simulink model "RajamaniController"  (R2018a)
settings: Solver=ode45  StartTime=0.0  StopTime=1  FixedStep=0.002  RelTol=1e-3  EnableMultiTasking=on
values from neighbouring files (symbols this model uses):
  A = [0 1 0 0; 0 A22 A23 A24; 0 0 0 1; 0 A42 A43 A44;]    [data.m]
  B1 = [0; B1_12; 0; B1_14]    [data.m]
  B2 = [0; B2_12; 0; B2_14]    [data.m]
  delta_ff = (L/R)+((Kv*ay)-(k3*e2_ss))    [data.m]
  K = place(A, B1, P)    [data.m]
  m = 1573    [data.m]
  PsiDot_des = Vx/R    (= 0.03)    [data.m]
undefined symbols (not defined in the file or in its folder): Bx_ash_f, Bx_ash_r, Bx_snow_f, Bx_snow_r, By_ash_f, By_ash_r, By_snow_f, By_snow_r, Cx_ash_f, Cx_ash_r, Cx_snow_f, Cx_snow_r, Cy_ash_f, Cy_ash_r, Cy_snow_f, Cy_snow_r, D_phi, D_theta, DELTA_OFFSET, delta_r, epsilon, Ex_ash_f, Ex_ash_r, Ex_snow_f, Ex_snow_r, Ey_ash_f, Ey_ash_r, Ey_snow_f, Ey_snow_r, g, h, Iw, Ixx, Iyy, Izz, K_phi, K_theta, l_f, l_r, mu_x_ash_f, mu_x_ash_r, mu_x_snow_f, mu_x_snow_r, mu_y_ash_f, mu_y_ash_r, mu_y_snow_f, mu_y_snow_r, omega0, road, Rw, Ts, Tsmall, Vx0, w
(part 2 of 2)

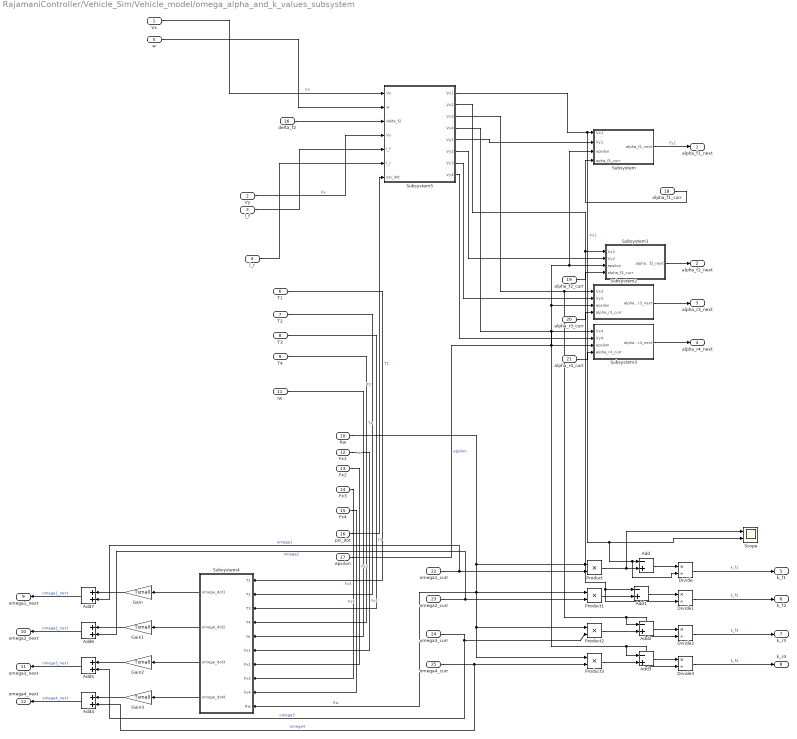
== system RajamaniController/Vehicle_Sim/Vehicle_model/omega_alpha_and_k_values_subsystem ==
  Vx : Inport  OutDataTypeStr=double  SampleTime=Ts
  Vy : Inport  Port=2  OutDataTypeStr=double  SampleTime=Ts
  l_f : Inport  Port=3  OutDataTypeStr=double  SampleTime=Ts
  l_r : Inport  Port=4  OutDataTypeStr=double  SampleTime=Ts
  w : Inport  Port=5  OutDataTypeStr=double  SampleTime=Ts
  T1 : Inport  Port=6  OutDataTypeStr=double  SampleTime=Ts
  T2 : Inport  Port=7  OutDataTypeStr=double  SampleTime=Ts
  T3 : Inport  Port=8  OutDataTypeStr=double  SampleTime=Ts
  T4 : Inport  Port=9  OutDataTypeStr=double  SampleTime=Ts
  Rw : Inport  Port=10  OutDataTypeStr=double  SampleTime=Ts
  Iw : Inport  Port=11  OutDataTypeStr=double  SampleTime=Ts
  Fx1 : Inport  Port=12  OutDataTypeStr=double  SampleTime=Ts
  Fx2 : Inport  Port=13  OutDataTypeStr=double  SampleTime=Ts
  Fx3 : Inport  Port=14  OutDataTypeStr=double  SampleTime=Ts
  Fx4 : Inport  Port=15  OutDataTypeStr=double  SampleTime=Ts
  psi_dot : Inport  Port=16  OutDataTypeStr=double  SampleTime=Ts
  epsilon : Inport  Port=17  OutDataTypeStr=double  SampleTime=Ts
  alpha_f1_curr : Inport  Port=18  OutDataTypeStr=double  SampleTime=Tsmall
  alpha_f2_curr : Inport  Port=19  OutDataTypeStr=double  SampleTime=Tsmall
  alpha_r3_curr : Inport  Port=20  OutDataTypeStr=double  SampleTime=Tsmall
  alpha_r4_curr : Inport  Port=21  OutDataTypeStr=double  SampleTime=Tsmall
  omega1_curr : Inport  Port=22  OutDataTypeStr=double  SampleTime=Ts
  omega2_curr : Inport  Port=23  OutDataTypeStr=double  SampleTime=Ts
  omega3_curr : Inport  Port=24  OutDataTypeStr=double  SampleTime=Ts
  omega4_curr : Inport  Port=25  OutDataTypeStr=double  SampleTime=Ts
  delta_f2 : Inport  Port=26  OutDataTypeStr=double  SampleTime=Ts
  Add{,1..3} (4 alike) : Sum  Inputs=-+
  Add{4..7} (4 alike) : Sum
  Divide{,1..3} (4 alike) : Product  Inputs=*/
  Gain{,1..3} (4 alike) : Gain  Gain=Tsmall
  Product{,1..3} (4 alike) : Product
  Scope : Scope  NumInputPorts=2
  Subsystem : Subsystem
  Subsystem1 : Subsystem
  Subsystem2 : Subsystem
  Subsystem3 : Subsystem
  Subsystem4 : Subsystem
  Subsystem5 : Subsystem
  alpha_f1_next : Outport  OutDataTypeStr=double  SampleTime=Ts
  alpha_f2_next : Outport  Port=2  OutDataTypeStr=double  SampleTime=Tsmall
  alpha_r3_next : Outport  Port=3  OutDataTypeStr=double  SampleTime=Tsmall
  alpha_r4_next : Outport  Port=4  OutDataTypeStr=double  SampleTime=Tsmall
  k_f1 : Outport  Port=5  OutDataTypeStr=double  SampleTime=Ts
  k_f2 : Outport  Port=6  OutDataTypeStr=double  SampleTime=Ts
  k_r3 : Outport  Port=7  OutDataTypeStr=double  SampleTime=Ts
  k_r4 : Outport  Port=8  OutDataTypeStr=double  SampleTime=Ts
  omega1_next : Outport  Port=9
  omega2_next : Outport  Port=10
  omega3_next : Outport  Port=11
  omega4_next : Outport  Port=12
  wires:
  Subsystem5/1(Vx1) -> Scope/2, Divide/2, Add/1, Subsystem/1(Vx1)  "Vx1"
  epsilon/1 -> Subsystem3/3(epsilon), Subsystem2/3(epsilon), Subsystem1/3(epsilon), Subsystem/3(epsilon)  "epsilon"
  Subsystem1/1(alpha_f2_next) -> alpha_f2_next/1
  Divide/1 -> k_f1/1  "k_f1"
  omega1_curr/1 -> Add7/2, Product/2  "omega1"
  omega2_curr/1 -> Add6/2, Product1/2  "omega2"
  omega3_curr/1 -> Add5/2, Product2/2  "omega3"
  omega4_curr/1 -> Add4/2, Product3/2  "omega4"
  Rw/1 -> Subsystem4/10(Rw), Product1/1, Product3/1, Product2/1, Product/1  "Rw"
  Product/1 -> Scope/1, Add/2
  Add/1 -> Divide/1
  Product1/1 -> Add1/2
  Add1/1 -> Divide1/1
  Product2/1 -> Add2/2
  Add2/1 -> Divide2/1
  Product3/1 -> Add3/2
  Add3/1 -> Divide3/1
  Divide1/1 -> k_f2/1  "k_f2"
  Divide2/1 -> k_r3/1  "k_f3"
  Divide3/1 -> k_r4/1  "k_f4"
  T1/1 -> Subsystem4/1(T1)  "T1"
  T2/1 -> Subsystem4/2(T2)  "T2"
  T3/1 -> Subsystem4/3(T3)  "T3"
  T4/1 -> Subsystem4/4(T4)  "T4"
  Iw/1 -> Subsystem4/5(Iw)  "Iw"
  Fx1/1 -> Subsystem4/6(Fx1)  "Fx1"
  Fx2/1 -> Subsystem4/7(Fx2)  "Fx2"
  Fx3/1 -> Subsystem4/8(Fx3)  "Fx3"
  Fx4/1 -> Subsystem4/9(Fx4)  "Fx4"
  Subsystem4/1(omega_dot1) -> Gain/1
  Subsystem4/2(omega_dot2) -> Gain1/1
  Subsystem4/3(omega_dot3) -> Gain2/1
  Subsystem4/4(omega_dot4) -> Gain3/1
  alpha_f1_curr/1 -> Subsystem/4(apha_f1_curr)
  alpha_f2_curr/1 -> Subsystem1/4(alpha_f2_curr)
  Subsystem2/1(alpha_r3_next) -> alpha_r3_next/1
  alpha_r3_curr/1 -> Subsystem2/4(alpha_r3_curr)
  Subsystem3/1(alpha_r4_next) -> alpha_r4_next/1
  alpha_r4_curr/1 -> Subsystem3/4(alpha_r4_curr)
  Gain1/1 -> Add6/1
  Gain/1 -> Add7/1
  Gain2/1 -> Add5/1
  Gain3/1 -> Add4/1
  Add7/1 -> omega1_next/1  "omega1_next"
  Add6/1 -> omega2_next/1  "omega2_next"
  Add5/1 -> omega3_next/1  "omega3_next"
  Add4/1 -> omega4_next/1  "omega4_next"
  Subsystem5/2(Vx2) -> Divide1/2, Add1/1, Subsystem1/1(Vx2)
  Subsystem5/4(Vx4) -> Subsystem3/1(Vx4), Add3/1, Divide3/2
  Subsystem5/3(Vx3) -> Subsystem2/1(Vx3), Add2/1, Divide2/2
  Vx/1 -> Subsystem5/1(Vx)  "Vx"
  w/1 -> Subsystem5/2(w)
  Vy/1 -> Subsystem5/4(Vy)  "Vy"
  l_f/1 -> Subsystem5/5(l_f)
  l_r/1 -> Subsystem5/6(l_r)
  psi_dot/1 -> Subsystem5/7(psi_dot)
  Subsystem5/5(Vy1) -> Subsystem/2(Vy1)
  Subsystem5/6(Vy2) -> Subsystem1/2(Vy2)
  Subsystem5/7(Vy3) -> Subsystem2/2(Vy3)
  Subsystem5/8(Vy4) -> Subsystem3/2(Vy4)
  delta_f2/1 -> Subsystem5/3(delta_f2)
  Subsystem/1(alpha_f1_next) -> alpha_f1_next/1  "Fy1"

== system RajamaniController/Vehicle_Sim/Vehicle_model/phi_subsystem ==
  FY : Inport  OutDataTypeStr=double  SampleTime=Ts
  psi_dot : Inport  Port=2  OutDataTypeStr=double  SampleTime=Tsmall
  phi_dot : Inport  Port=3  OutDataTypeStr=double  SampleTime=Tsmall
  phi : Inport  Port=4  OutDataTypeStr=double  SampleTime=Tsmall
  theta_dot : Inport  Port=5  OutDataTypeStr=double  SampleTime=Tsmall
  theta : Inport  Port=6  OutDataTypeStr=double  SampleTime=Tsmall
  Ixx : Inport  Port=7  OutDataTypeStr=double  SampleTime=Ts
  Iyy : Inport  Port=8  OutDataTypeStr=double  SampleTime=Ts
  Izz : Inport  Port=9  OutDataTypeStr=double  SampleTime=Ts
  K_phi : Inport  Port=10  OutDataTypeStr=double  SampleTime=Ts
  D_phi : Inport  Port=11  OutDataTypeStr=double  SampleTime=Ts
  h : Inport  Port=12  OutDataTypeStr=double  SampleTime=Ts
  Divide : Product  Inputs=*/
  phi_ddot_denominator_subsystem : Subsystem
  phi_ddot_numerator_subsystem : Subsystem
  phi_ddot : Outport  OutDataTypeStr=double  SampleTime=Tsmall
  wires:
  phi_ddot_numerator_subsystem/1(phi_ddot_numerator) -> Divide/1
  phi/1 -> phi_ddot_denominator_subsystem/1(phi), phi_ddot_numerator_subsystem/4(phi)
  FY/1 -> phi_ddot_numerator_subsystem/1(FY)
  theta_dot/1 -> phi_ddot_numerator_subsystem/5(theta_dot)
  phi_dot/1 -> phi_ddot_numerator_subsystem/3(phi_dot)
  theta/1 -> phi_ddot_numerator_subsystem/6(theta), phi_ddot_denominator_subsystem/2(theta)
  psi_dot/1 -> phi_ddot_numerator_subsystem/2(psi_dot)
  Divide/1 -> phi_ddot/1
  phi_ddot_denominator_subsystem/1(phi_ddot_denominator) -> Divide/2
  Ixx/1 -> phi_ddot_denominator_subsystem/3(Ixx)
  Iyy/1 -> phi_ddot_denominator_subsystem/4(Iyy), phi_ddot_numerator_subsystem/7(Iyy)
  Izz/1 -> phi_ddot_numerator_subsystem/8(Izz), phi_ddot_denominator_subsystem/5(Izz)
  K_phi/1 -> phi_ddot_numerator_subsystem/9(K_phi)
  D_phi/1 -> phi_ddot_numerator_subsystem/10(D_phi)
  h/1 -> phi_ddot_numerator_subsystem/11(h)

== system RajamaniController/Vehicle_Sim/Vehicle_model/psi_subsystem ==
  FX : Inport  OutDataTypeStr=double  SampleTime=Ts
  FY : Inport  Port=2  OutDataTypeStr=double  SampleTime=Ts
  MZ : Inport  Port=3  OutDataTypeStr=double  SampleTime=Ts
  phi : Inport  Port=4  OutDataTypeStr=double  SampleTime=Ts
  theta : Inport  Port=5  OutDataTypeStr=double  SampleTime=Ts
  Ixx : Inport  Port=6  OutDataTypeStr=double  SampleTime=Ts
  Iyy : Inport  Port=7  OutDataTypeStr=double  SampleTime=Ts
  Izz : Inport  Port=8  OutDataTypeStr=double  SampleTime=Ts
  h : Inport  Port=9  OutDataTypeStr=double  SampleTime=Ts
  Add : Sum
  Add1 : Sum  Inputs=+-
  Add2 : Sum
  Add3 : Sum
  Divide{,1..6,8} (8 alike) : Product  Inputs=**
  Divide7 : Product  Inputs=*/
  Square{,1..3} (4 alike) : Math  Operator=square  RndMeth=Zero  SaturateOnIntegerOverflow=on
  Trigonometric Function : Trigonometry
  Trigonometric Function1 : Trigonometry
  Trigonometric Function2 : Trigonometry  Operator=cos
  Trigonometric Function3 : Trigonometry  Operator=cos
  psi_ddot : Outport
  wires:
  Square/1 -> Divide3/1
  MZ/1 -> Add1/1
  Trigonometric Function2/1 -> Square2/1, Divide2/1
  Divide2/1 -> Add/2
  Ixx/1 -> Divide3/2
  Add2/1 -> Divide4/2
  Square2/1 -> Divide6/2
  Divide6/1 -> Add2/2
  Divide3/1 -> Add3/1
  Add3/1 -> Divide7/2
  FY/1 -> Divide1/1
  FX/1 -> Divide/1
  Trigonometric Function3/1 -> Square3/1
  Iyy/1 -> Divide5/1
  Divide1/1 -> Divide2/2
  Square3/1 -> Divide4/1
  Izz/1 -> Divide6/1
  Trigonometric Function/1 -> Square/1, Divide1/2
  Trigonometric Function1/1 -> Square1/1, Divide/2
  phi/1 -> Trigonometric Function1/1, Trigonometric Function2/1
  theta/1 -> Trigonometric Function3/1, Trigonometric Function/1
  Divide8/1 -> Add1/2
  Add/1 -> Divide8/1
  Divide5/1 -> Add2/1
  Add1/1 -> Divide7/1
  Divide/1 -> Add/1
  Divide7/1 -> psi_ddot/1  "psi_ddot"
  Divide4/1 -> Add3/2
  Square1/1 -> Divide5/2
  h/1 -> Divide8/2

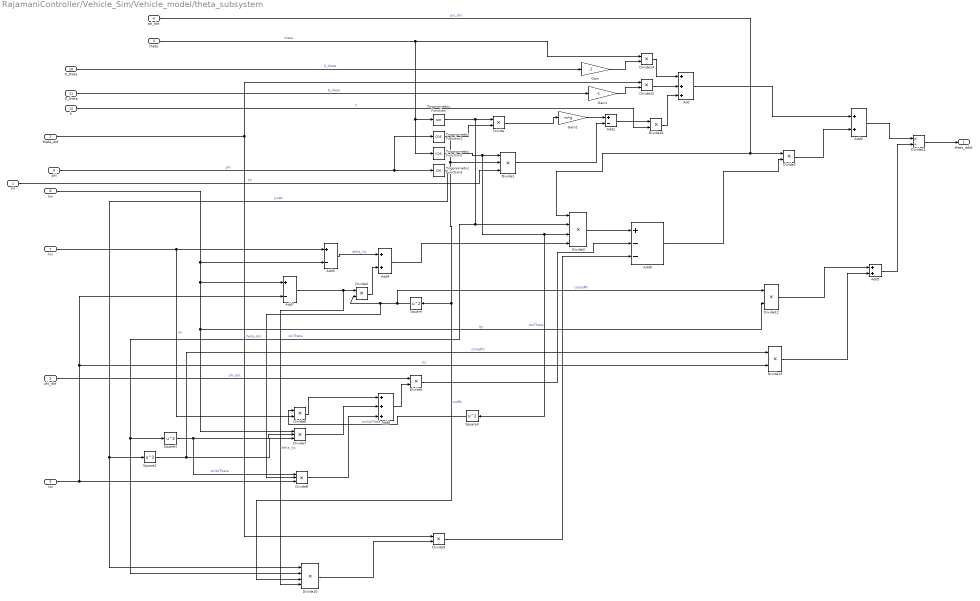
== system RajamaniController/Vehicle_Sim/Vehicle_model/theta_subsystem ==
  FX : Inport  OutDataTypeStr=double  SampleTime=Ts
  theta_dot : Inport  Port=2  OutDataTypeStr=double  SampleTime=Ts
  theta : Inport  Port=3  OutDataTypeStr=double  SampleTime=Ts
  psi_dot : Inport  Port=4  OutDataTypeStr=double  SampleTime=Ts
  phi_dot : Inport  Port=5  OutDataTypeStr=double  SampleTime=Ts
  phi : Inport  Port=6  OutDataTypeStr=double  SampleTime=Ts
  Ixx : Inport  Port=7  OutDataTypeStr=double  SampleTime=Ts
  Iyy : Inport  Port=8  OutDataTypeStr=double  SampleTime=Ts
  Izz : Inport  Port=9  OutDataTypeStr=double  SampleTime=Ts
  K_theta : Inport  Port=10  OutDataTypeStr=double  SampleTime=Ts
  D_theta : Inport  Port=11  OutDataTypeStr=double  SampleTime=Ts
  h : Inport  Port=12  OutDataTypeStr=double  SampleTime=Ts
  Add : Sum  Inputs=+++
  Add1 : Sum  Inputs=+-
  Add2 : Sum
  Add3 : Sum  Inputs=+-
  Add4 : Sum
  Add5 : Sum
  Add7 : Sum  Inputs=+-
  Add8 : Sum  Inputs=+++
  Add9 : Sum  Inputs=+--
  Divide{,2,4..6,9,12..16} (11 alike) : Product  Inputs=**
  Divide1 : Product  Inputs=***
  Divide10 : Product  Inputs=****
  Divide11 : Product  Inputs=*/
  Divide3 : Product  Inputs=****
  Divide7 : Product  Inputs=***
  Divide8 : Product  Inputs=***
  Gain : Gain  Gain=-1  OutDataTypeStr=double
  Gain1 : Gain  Gain=-1  OutDataTypeStr=double
  Gain2 : Gain  Gain=m*g  OutDataTypeStr=double
  Square{,1..3} (4 alike) : Math  Operator=square  RndMeth=Zero  SaturateOnIntegerOverflow=on
  Trigonometric Function : Trigonometry
  Trigonometric Function1 : Trigonometry  Operator=cos
  Trigonometric Function2 : Trigonometry  Operator=cos
  Trigonometric Function3 : Trigonometry
  theta_ddot : Outport  OutDataTypeStr=double  SampleTime=Tsmall
  wires:
  Add/1 -> Add2/1
  Divide8/1 -> Add8/3
  Add4/1 -> Divide3/4
  Divide1/1 -> Add1/2
  Add8/1 -> Divide5/2
  Add1/1 -> Divide16/1
  Square1/1 -> Divide8/1, Divide7/2  "sinSqTheta"
  Divide7/1 -> Add8/2
  Add9/1 -> Divide2/2
  Square/1 -> Divide12/1, Divide8/2, Divide4/2  "cosSqPhi"
  Trigonometric Function3/1 -> Divide10/1, Square2/1  "sinPhi"
  Gain2/1 -> Add1/1
  Square2/1 -> Divide13/1, Divide7/3  "sinSqPhi"
  Trigonometric Function2/1 -> Square3/1, Divide3/3, Divide1/1  "cosTheta"
  Divide/1 -> Gain2/1
  Divide10/1 -> Divide9/2
  Trigonometric Function/1 -> Divide10/2, Square1/1, Divide3/2, Divide/1  "sinTheta"
  Divide6/1 -> Add8/1
  Divide2/1 -> Add2/2
  Divide9/1 -> Add9/3
  Divide5/1 -> Add9/2
  Gain/1 -> Divide14/2
  Divide4/1 -> Add4/2
  Add3/1 -> Add4/1  "delta_Ixy"
  Divide3/1 -> Add9/1
  Trigonometric Function1/1 -> Divide10/3, Square/1, Divide1/2, Divide/2  "cosPhi"
  Add7/1 -> Divide10/4, Divide4/1  "delta_Iyz"
  Divide16/1 -> Add/3
  Gain1/1 -> Divide15/2
  theta/1 -> Divide14/1, Trigonometric Function/1, Trigonometric Function2/1  "theta"
  Iyy/1 -> Divide7/1, Divide12/2, Add7/1, Add3/2  "Iyy"
  phi_dot/1 -> Divide5/1  "phi_dot"
  Ixx/1 -> Add3/1, Divide6/2  "Ixx"
  FX/1 -> Divide1/3  "FX"
  theta_dot/1 -> Divide15/1, Divide9/1  "theta_dot"
  Izz/1 -> Divide13/2, Add7/2, Divide8/3  "Izz"
  phi/1 -> Trigonometric Function1/1, Trigonometric Function3/1  "phi"
  psi_dot/1 -> Divide3/1, Divide2/1  "psi_dot"
  Add2/1 -> Divide11/1
  Divide11/1 -> theta_ddot/1
  Add5/1 -> Divide11/2
  Divide12/1 -> Add5/1
  Divide13/1 -> Add5/2
  Divide15/1 -> Add/2
  Divide14/1 -> Add/1
  K_theta/1 -> Gain/1  "K_theta"
  D_theta/1 -> Gain1/1  "D_theta"
  h/1 -> Divide16/2  "h"
  Square3/1 -> Divide6/1  "cosSqTheta"

== system RajamaniController/Vehicle_Sim/Vehicle_model/Fz_Subsystem/tau_phi_subsystem ==
  K_phi : Inport
  D_phi : Inport  Port=2
  phi_dot : Inport  Port=3
  phi : Inport  Port=4
  Add : Sum
  Add1 : Sum
  Divide{,1..3} (4 alike) : Product  Inputs=**
  Gain : Gain  Gain=0.5
  Gain1 : Gain  Gain=0.5
  tau_phi_f : Outport
  tau_phi_r : Outport  Port=2
  wires:
  Divide2/1 -> Add1/1
  Divide/1 -> Add/1
  Add/1 -> tau_phi_f/1  "tau_phi_f"
  Divide1/1 -> Add/2
  Gain1/1 -> Divide3/1, Divide1/1  "D_phi_r"
  Gain/1 -> Divide2/1, Divide/1  "K_phi_r"
  D_phi/1 -> Gain1/1
  phi/1 -> Divide2/2, Divide/2  "phi"
  Divide3/1 -> Add1/2
  phi_dot/1 -> Divide3/2, Divide1/2  "phi_dot"
  K_phi/1 -> Gain/1
  Add1/1 -> tau_phi_r/1  "tau_phi_r"

== system RajamaniController/Vehicle_Sim/Vehicle_model/Fz_Subsystem/tau_theta_subsystem ==
  theta_dot : Inport  OutDataTypeStr=double  SampleTime=Ts  LockScale=on
  theta : Inport  Port=2  OutDataTypeStr=double  SampleTime=Ts
  K_theta : Inport  Port=3  OutDataTypeStr=double  SampleTime=Ts
  D_theta : Inport  Port=4  OutDataTypeStr=double  SampleTime=Ts
  Add : Sum
  Divide : Product  Inputs=**
  Divide1 : Product  Inputs=**
  tau_theta : Outport  OutDataTypeStr=double  SampleTime=Ts
  wires:
  Add/1 -> tau_theta/1
  Divide/1 -> Add/1
  Divide1/1 -> Add/2
  K_theta/1 -> Divide/1
  D_theta/1 -> Divide1/2
  theta_dot/1 -> Divide1/1
  theta/1 -> Divide/2

== system RajamaniController/Vehicle_Sim/Vehicle_model/Pacjeka_parameters_Subsystem/Ashphalt_condition_subsystem ==
  Action Port : ActionPort
  Bx_ash_f : Constant  Value=Bx_ash_f
  Bx_ash_r : Constant  Value=Bx_ash_r
  By_ash_f : Constant  Value=By_ash_f
  By_ash_r : Constant  Value=By_ash_r
  Cx_ash_f : Constant  Value=Cx_ash_f
  Cx_ash_r : Constant  Value=Cx_ash_r
  Cy_ash_f : Constant  Value=Cy_ash_f
  Cy_ash_r : Constant  Value=Cy_ash_r
  Ex_ash_f : Constant  Value=Ex_ash_f
  Ex_ash_r : Constant  Value=Ex_ash_r
  Ey_ash_f : Constant  Value=Ey_ash_f
  Ey_ash_r : Constant  Value=Ey_ash_r
  Mux : Mux  Inputs=16
      settings: DisplayOption=signals
  mu_x_ash_f : Constant  Value=mu_x_ash_f
  mu_x_ash_r : Constant  Value=mu_x_ash_r
  mu_y_ash_f : Constant  Value=mu_y_ash_f
  mu_y_ash_r : Constant  Value=mu_y_ash_r
  Out1 : Outport  OutDataTypeStr=double  SampleTime=Ts
  wires:
  mu_x_ash_f/1 -> Mux/1  "mu_x_ash_f"
  mu_y_ash_f/1 -> Mux/2  "mu_y_ash_f"
  Cx_ash_f/1 -> Mux/3  "Cx_ash_f"
  Cy_ash_f/1 -> Mux/4  "Cy_ash_f"
  Bx_ash_f/1 -> Mux/5  "Bx_ash_f"
  By_ash_f/1 -> Mux/6  "By_ash_f"
  Ex_ash_f/1 -> Mux/7  "Ex_ash_f"
  Ey_ash_f/1 -> Mux/8  "E_y_ash_f"
  Cy_ash_r/1 -> Mux/12  "Cy_ash_r"
  Cx_ash_r/1 -> Mux/11  "Cx_ash_r"
  By_ash_r/1 -> Mux/14  "By_ash_r"
  Bx_ash_r/1 -> Mux/13  "Bx_ash_r"
  mu_y_ash_r/1 -> Mux/10  "mu_y_ash_r"
  Ex_ash_r/1 -> Mux/15  "Ex_ash_r"
  mu_x_ash_r/1 -> Mux/9  "mu_x_ash_r"
  Ey_ash_r/1 -> Mux/16  "Ey_ash_r"
  Mux/1 -> Out1/1

== system RajamaniController/Vehicle_Sim/Vehicle_model/Pacjeka_parameters_Subsystem/Snow_condition_subsystem ==
  Action Port : ActionPort
  Bx_snow_f : Constant  Value=Bx_snow_f
  Bx_snow_r : Constant  Value=Bx_snow_r
  By_snow_f : Constant  Value=By_snow_f
  By_snow_r : Constant  Value=By_snow_r
  Cx_snow_f : Constant  Value=Cx_snow_f
  Cx_snow_r : Constant  Value=Cx_snow_r
  Cy_snow_f : Constant  Value=Cy_snow_f
  Cy_snow_r : Constant  Value=Cy_snow_r
  Ex_snow_f : Constant  Value=Ex_snow_f
  Ex_snow_r : Constant  Value=Ex_snow_r
  Ey_snow_f : Constant  Value=Ey_snow_f
  Ey_snow_r : Constant  Value=Ey_snow_r
  Mux : Mux  Inputs=16
  mu_x_snow_f : Constant  Value=mu_x_snow_f
  mu_x_snow_r : Constant  Value=mu_x_snow_r
  mu_y_snow_f : Constant  Value=mu_y_snow_f
  mu_y_snow_r : Constant  Value=mu_y_snow_r
  Out1 : Outport  OutDataTypeStr=double  SampleTime=Ts
  wires:
  Ex_snow_r/1 -> Mux/15
  Cy_snow_r/1 -> Mux/12
  By_snow_r/1 -> Mux/14
  Cx_snow_r/1 -> Mux/11
  mu_y_snow_r/1 -> Mux/10
  mu_x_snow_r/1 -> Mux/9
  Bx_snow_r/1 -> Mux/13
  Ey_snow_r/1 -> Mux/16
  mu_x_snow_f/1 -> Mux/1
  mu_y_snow_f/1 -> Mux/2
  Cx_snow_f/1 -> Mux/3
  Cy_snow_f/1 -> Mux/4
  Bx_snow_f/1 -> Mux/5
  By_snow_f/1 -> Mux/6
  Ex_snow_f/1 -> Mux/7
  Ey_snow_f/1 -> Mux/8
  Mux/1 -> Out1/1

== system RajamaniController/Vehicle_Sim/Vehicle_model/omega_alpha_and_k_values_subsystem/Subsystem ==
  Vx1 : Inport  OutDataTypeStr=double  SampleTime=Ts
  Vy1 : Inport  Port=2  OutDataTypeStr=double  SampleTime=Ts
  epsilon : Inport  Port=3  OutDataTypeStr=double  SampleTime=Ts
  apha_f1_curr : Inport  Port=4  OutDataTypeStr=double  SampleTime=Tsmall
  Add : Sum  Inputs=+-
  Add1 : Sum
  Divide : Product  Inputs=*/
  Divide1 : Product  Inputs=*/
  Gain : Gain  Gain=-1
  Gain1 : Gain  Gain=Tsmall
  Product : Product
  Product1 : Product
  Trigonometric Function : Trigonometry  Operator=atan
  alpha_f1_next : Outport  OutDataTypeStr=double  SampleTime=Tsmall
  wires:
  Gain1/1 -> Add1/1  "alpha_f1dot*Tsmall"
  Vx1/1 -> Divide1/2, Divide/1
  Product1/1 -> Add/2
  Divide1/1 -> Trigonometric Function/1
  Divide/1 -> Gain/1, Product1/1
  Product/1 -> Add/1
  epsilon/1 -> Divide/2
  Trigonometric Function/1 -> Product/2
  Vy1/1 -> Divide1/1
  Add/1 -> Gain1/1  "alpha_f1_dot"
  Gain/1 -> Product/1
  Add1/1 -> alpha_f1_next/1
  apha_f1_curr/1 -> Add1/2, Product1/2  "Fy1"

== system RajamaniController/Vehicle_Sim/Vehicle_model/omega_alpha_and_k_values_subsystem/Subsystem1 ==
  Vx2 : Inport  OutDataTypeStr=double  SampleTime=Ts
  Vy2 : Inport  Port=2  OutDataTypeStr=double  SampleTime=Ts
  epsilon : Inport  Port=3  OutDataTypeStr=double  SampleTime=Ts
  alpha_f2_curr : Inport  Port=4  OutDataTypeStr=double  SampleTime=Tsmall
  Add : Sum  Inputs=+-
  Add1 : Sum
  Divide : Product  Inputs=*/
  Divide1 : Product  Inputs=*/
  Gain : Gain  Gain=-1
  Gain1 : Gain  Gain=Tsmall
  Product : Product
  Product1 : Product
  Trigonometric Function : Trigonometry  Operator=atan
  alpha_f2_next : Outport  OutDataTypeStr=double  SampleTime=Tsmall
  wires:
  Gain1/1 -> Add1/1  "alpha_f2dot*Tsmall"
  Vx2/1 -> Divide1/2, Divide/1
  Product1/1 -> Add/2
  Divide1/1 -> Trigonometric Function/1
  Divide/1 -> Gain/1, Product1/1
  Product/1 -> Add/1
  epsilon/1 -> Divide/2
  Trigonometric Function/1 -> Product/2
  Vy2/1 -> Divide1/1
  Add/1 -> Gain1/1  "alpha_f2_dot"
  Gain/1 -> Product/1
  alpha_f2_curr/1 -> Add1/2, Product1/2
  Add1/1 -> alpha_f2_next/1

== system RajamaniController/Vehicle_Sim/Vehicle_model/omega_alpha_and_k_values_subsystem/Subsystem2 ==
  Vx3 : Inport  OutDataTypeStr=double  SampleTime=Ts
  Vy3 : Inport  Port=2  OutDataTypeStr=double  SampleTime=Ts
  epsilon : Inport  Port=3  OutDataTypeStr=double  SampleTime=Ts
  alpha_r3_curr : Inport  Port=4  OutDataTypeStr=double  SampleTime=Tsmall
  Add : Sum  Inputs=+-
  Add1 : Sum
  Divide : Product  Inputs=*/
  Divide1 : Product  Inputs=*/
  Gain : Gain  Gain=-1
  Gain1 : Gain  Gain=Tsmall
  Product : Product
  Product1 : Product
  Trigonometric Function : Trigonometry  Operator=atan
  alpha_r3_next : Outport  OutDataTypeStr=double  SampleTime=Tsmall
  wires:
  Gain1/1 -> Add1/1  "alpha_r3dot*Tsmall"
  Vx3/1 -> Divide1/2, Divide/1
  Product1/1 -> Add/2
  Divide1/1 -> Trigonometric Function/1
  Divide/1 -> Gain/1, Product1/1
  Product/1 -> Add/1
  epsilon/1 -> Divide/2
  Trigonometric Function/1 -> Product/2
  Vy3/1 -> Divide1/1
  Add/1 -> Gain1/1  "alpha_r3_dot"
  Gain/1 -> Product/1
  alpha_r3_curr/1 -> Add1/2, Product1/2
  Add1/1 -> alpha_r3_next/1

== system RajamaniController/Vehicle_Sim/Vehicle_model/omega_alpha_and_k_values_subsystem/Subsystem3 ==
  Vx4 : Inport  OutDataTypeStr=double  SampleTime=Ts
  Vy4 : Inport  Port=2  OutDataTypeStr=double  SampleTime=Ts
  epsilon : Inport  Port=3  OutDataTypeStr=double  SampleTime=Ts
  alpha_r4_curr : Inport  Port=4  OutDataTypeStr=double  SampleTime=Tsmall
  Add : Sum  Inputs=+-
  Add1 : Sum
  Divide : Product  Inputs=*/
  Divide1 : Product  Inputs=*/
  Gain : Gain  Gain=-1
  Gain1 : Gain  Gain=Tsmall
  Product : Product
  Product1 : Product
  Trigonometric Function : Trigonometry  Operator=atan
  alpha_r4_next : Outport  OutDataTypeStr=double  SampleTime=Tsmall
  wires:
  Gain1/1 -> Add1/1  "alpha_r4dot*Tsmall"
  Vx4/1 -> Divide1/2, Divide/1
  Product1/1 -> Add/2
  Divide1/1 -> Trigonometric Function/1
  Divide/1 -> Gain/1, Product1/1
  Product/1 -> Add/1
  epsilon/1 -> Divide/2
  Trigonometric Function/1 -> Product/2
  Vy4/1 -> Divide1/1
  Add/1 -> Gain1/1  "alpha_r4_dot"
  Gain/1 -> Product/1
  alpha_r4_curr/1 -> Add1/2, Product1/2
  Add1/1 -> alpha_r4_next/1

== system RajamaniController/Vehicle_Sim/Vehicle_model/omega_alpha_and_k_values_subsystem/Subsystem4 ==
  T1 : Inport  OutDataTypeStr=double  SampleTime=Ts
  T2 : Inport  Port=2  OutDataTypeStr=double  SampleTime=Ts
  T3 : Inport  Port=3  OutDataTypeStr=double  SampleTime=Ts
  T4 : Inport  Port=4  OutDataTypeStr=double  SampleTime=Ts
  Iw : Inport  Port=5  OutDataTypeStr=double  SampleTime=Ts
  Fx1 : Inport  Port=6  OutDataTypeStr=double  SampleTime=Ts
  Fx2 : Inport  Port=7  OutDataTypeStr=double  SampleTime=Ts
  Fx3 : Inport  Port=8  OutDataTypeStr=double  SampleTime=Ts
  Fx4 : Inport  Port=9  OutDataTypeStr=double  SampleTime=Ts
  Rw : Inport  Port=10  OutDataTypeStr=double  SampleTime=Ts
  Add{4..7} (4 alike) : Sum  Inputs=+-
  Divide{4..7} (4 alike) : Product  Inputs=*/
  Product{4..7} (4 alike) : Product
  omega_dot1 : Outport  OutDataTypeStr=double  SampleTime=Tsmall
  omega_dot2 : Outport  Port=2  OutDataTypeStr=double  SampleTime=Tsmall
  omega_dot3 : Outport  Port=3  OutDataTypeStr=double  SampleTime=Tsmall
  omega_dot4 : Outport  Port=4  OutDataTypeStr=double  SampleTime=Tsmall
  wires:
  Product7/1 -> Add7/2
  Add7/1 -> Divide7/1
  Iw/1 -> Divide7/2, Divide6/2, Divide5/2, Divide4/2
  Add5/1 -> Divide5/1
  T1/1 -> Add4/1
  Product5/1 -> Add5/2
  Rw/1 -> Product4/2, Product5/2, Product7/2, Product6/2
  Divide7/1 -> omega_dot4/1  "omega_dot4"
  Fx3/1 -> Product6/1
  Add4/1 -> Divide4/1
  Fx2/1 -> Product5/1
  T4/1 -> Add7/1
  Fx1/1 -> Product4/1
  T3/1 -> Add6/1
  Product4/1 -> Add4/2
  T2/1 -> Add5/1
  Product6/1 -> Add6/2
  Add6/1 -> Divide6/1
  Fx4/1 -> Product7/1
  Divide6/1 -> omega_dot3/1  "omega_dot3"
  Divide5/1 -> omega_dot2/1  "omega_dot2"
  Divide4/1 -> omega_dot1/1  "omega_dot1"

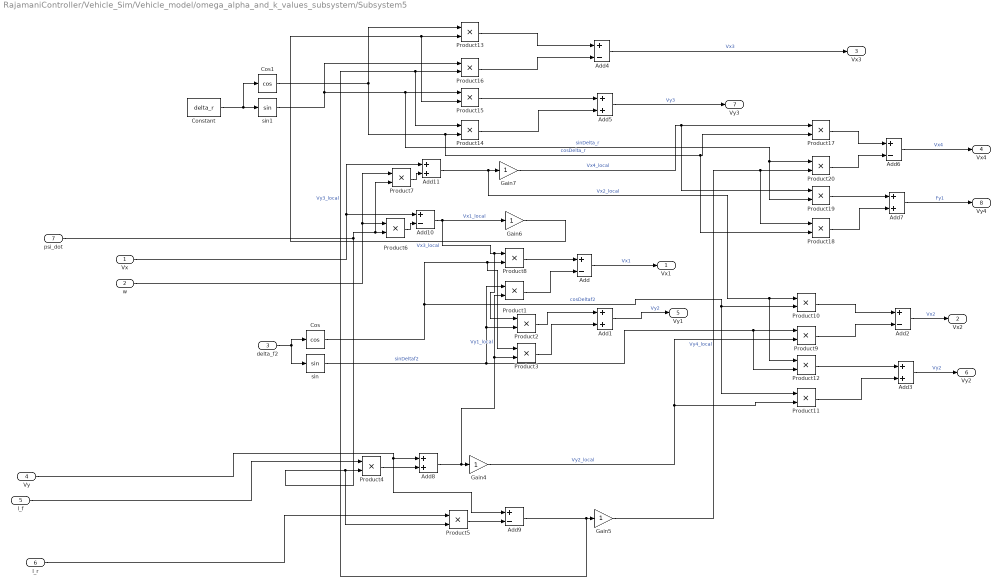
== system RajamaniController/Vehicle_Sim/Vehicle_model/omega_alpha_and_k_values_subsystem/Subsystem5 ==
  Vx : Inport  OutDataTypeStr=double  SampleTime=Ts
  w : Inport  Port=2  OutDataTypeStr=double  SampleTime=Ts
  delta_f2 : Inport  Port=3  OutDataTypeStr=double  SampleTime=Ts
  Vy : Inport  Port=4  OutDataTypeStr=double  SampleTime=Ts
  l_f : Inport  Port=5  OutDataTypeStr=double  SampleTime=Ts
  l_r : Inport  Port=6  OutDataTypeStr=double  SampleTime=Ts
  psi_dot : Inport  Port=7  OutDataTypeStr=double  SampleTime=Ts
  Add{,2,4,6,9..10} (6 alike) : Sum  Inputs=+-
  Add{1,3,5,7..8,11} (6 alike) : Sum
  Constant : Constant  Value=delta_r
  Cos : Trigonometry  Operator=cos
  Cos1 : Trigonometry  Operator=cos
  Gain{4..7} (4 alike) : Gain
  Product{1..20} (20 alike) : Product
  sin : Trigonometry
  sin1 : Trigonometry
  Vx1 : Outport  OutDataTypeStr=double  SampleTime=Ts
  Vx2 : Outport  Port=2  OutDataTypeStr=double  SampleTime=Ts
  Vx3 : Outport  Port=3  OutDataTypeStr=double  SampleTime=Ts
  Vx4 : Outport  Port=4  OutDataTypeStr=double  SampleTime=Ts
  Vy1 : Outport  Port=5  OutDataTypeStr=double  SampleTime=Ts
  Vy2 : Outport  Port=6  OutDataTypeStr=double  SampleTime=Ts
  Vy3 : Outport  Port=7  OutDataTypeStr=double  SampleTime=Ts
  Vy4 : Outport  Port=8  OutDataTypeStr=double  SampleTime=Ts
  wires:
  Product6/1 -> Add10/2
  Product7/1 -> Add11/2
  Gain7/1 -> Product19/1, Product17/1  "Vx4_local"
  Add11/1 -> Product10/1, Product12/1, Gain7/1  "Vx2_local"
  Gain6/1 -> Product15/2, Product13/2  "Vx3_local"
  w/1 -> Product6/1, Product7/1
  psi_dot/1 -> Product7/2, Product6/2, Product5/2, Product4/2
  Add10/1 -> Product2/1, Product8/1, Gain6/1  "Vx1_local"
  Add8/1 -> Product3/2, Product1/2, Gain4/1  "Vy1_local"
  l_f/1 -> Product4/1
  Product5/1 -> Add9/2
  Gain5/1 -> Product18/1, Product20/2  "Vy4_local"
  Product4/1 -> Add8/2
  Gain4/1 -> Product9/2, Product11/2  "Vy2_local"
  l_r/1 -> Product5/1
  Add9/1 -> Product14/1, Product16/2, Gain5/1  "Vy3_local"
  Vy/1 -> Add9/1, Add8/1
  Vx/1 -> Add10/1, Add11/1
  Cos/1 -> Product3/1, Product8/2, Product11/1, Product10/2  "cosDeltaf2"
  Product8/1 -> Add/1
  delta_f2/1 -> Cos/1, sin/1
  sin/1 -> Product12/2, Product9/1, Product1/1, Product2/2  "sinDeltaf2"
  Product1/1 -> Add/2
  Add/1 -> Vx1/1  "Vx1"
  Product2/1 -> Add1/1
  Product3/1 -> Add1/2
  Add1/1 -> Vy1/1  "Vy2"
  Product12/1 -> Add3/1
  Product11/1 -> Add3/2
  Product10/1 -> Add2/1
  Product9/1 -> Add2/2
  Add2/1 -> Vx2/1  "Vx2"
  Add3/1 -> Vy2/1  "Vy2"
  Constant/1 -> Cos1/1, sin1/1
  Cos1/1 -> Product18/2, Product17/2, Product14/2, Product13/1  "cosDelta_r"
  sin1/1 -> Product19/2, Product20/1, Product15/1, Product16/1  "sinDelta_r"
  Product15/1 -> Add5/1
  Product14/1 -> Add5/2
  Product13/1 -> Add4/1
  Product16/1 -> Add4/2
  Add4/1 -> Vx3/1  "Vx3"
  Add5/1 -> Vy3/1  "Vy3"
  Product17/1 -> Add6/1
  Product20/1 -> Add6/2
  Add6/1 -> Vx4/1  "Vx4"
  Product19/1 -> Add7/1
  Product18/1 -> Add7/2
  Add7/1 -> Vy4/1  "Fy1"

== system RajamaniController/Vehicle_Sim/Vehicle_model/phi_subsystem/phi_ddot_denominator_subsystem ==
  phi : Inport  OutDataTypeStr=double  SampleTime=Tsmall
  theta : Inport  Port=2  OutDataTypeStr=double  SampleTime=Tsmall
  Ixx : Inport  Port=3  OutDataTypeStr=double  SampleTime=Ts
  Iyy : Inport  Port=4  OutDataTypeStr=double  SampleTime=Ts
  Izz : Inport  Port=5  OutDataTypeStr=double  SampleTime=Ts
  Add : Sum  Inputs=+++
  Divide : Product  Inputs=**
  Divide1 : Product  Inputs=***
  Divide2 : Product  Inputs=***
  Square{,1..3} (4 alike) : Math  Operator=square  RndMeth=Zero  SaturateOnIntegerOverflow=on
  Trigonometric Function : Trigonometry  Operator=cos
  Trigonometric Function1 : Trigonometry
  Trigonometric Function2 : Trigonometry
  Trigonometric Function3 : Trigonometry  Operator=cos
  phi_ddot_denominator : Outport  OutDataTypeStr=double  SampleTime=Tsmall
  wires:
  Trigonometric Function1/1 -> Square1/1
  Iyy/1 -> Divide1/2
  Square1/1 -> Divide2/1, Divide1/1
  Square3/1 -> Divide2/2
  Square2/1 -> Divide1/3
  phi/1 -> Trigonometric Function2/1, Trigonometric Function3/1
  theta/1 -> Trigonometric Function1/1, Trigonometric Function/1
  Divide2/1 -> Add/3
  Divide/1 -> Add/1
  Add/1 -> phi_ddot_denominator/1
  Trigonometric Function3/1 -> Square3/1
  Izz/1 -> Divide2/3
  Square/1 -> Divide/1
  Trigonometric Function/1 -> Square/1
  Divide1/1 -> Add/2
  Ixx/1 -> Divide/2
  Trigonometric Function2/1 -> Square2/1

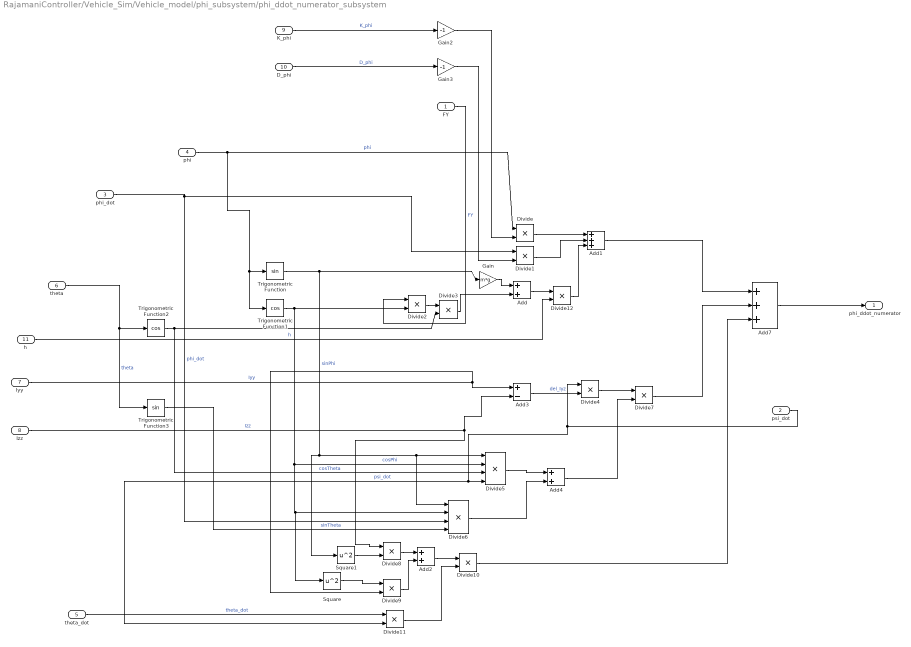
== system RajamaniController/Vehicle_Sim/Vehicle_model/phi_subsystem/phi_ddot_numerator_subsystem ==
  FY : Inport  OutDataTypeStr=double  SampleTime=Ts
  psi_dot : Inport  Port=2  OutDataTypeStr=double  SampleTime=Tsmall
  phi_dot : Inport  Port=3  OutDataTypeStr=double  SampleTime=Tsmall
  phi : Inport  Port=4  OutDataTypeStr=double  SampleTime=Tsmall
  theta_dot : Inport  Port=5  OutDataTypeStr=double  SampleTime=Tsmall
  theta : Inport  Port=6  OutDataTypeStr=double  SampleTime=Tsmall
  Iyy : Inport  Port=7  OutDataTypeStr=double  SampleTime=Ts
  Izz : Inport  Port=8  OutDataTypeStr=double  SampleTime=Ts
  K_phi : Inport  Port=9  OutDataTypeStr=double  SampleTime=Ts
  D_phi : Inport  Port=10  OutDataTypeStr=double  SampleTime=Ts
  h : Inport  Port=11  OutDataTypeStr=double  SampleTime=Ts
  Add : Sum
  Add1 : Sum  Inputs=+++
  Add2 : Sum
  Add3 : Sum  Inputs=+-
  Add4 : Sum
  Add7 : Sum  Inputs=+++
  Divide{,1..4,7..12} (11 alike) : Product  Inputs=**
  Divide5 : Product  Inputs=****
  Divide6 : Product  Inputs=****
  Gain : Gain  Gain=m*g
  Gain2 : Gain  Gain=-1
  Gain3 : Gain  Gain=-1
  Square : Math  Operator=square  RndMeth=Zero  SaturateOnIntegerOverflow=on
  Square1 : Math  Operator=square  RndMeth=Zero  SaturateOnIntegerOverflow=on
  Trigonometric Function : Trigonometry
  Trigonometric Function1 : Trigonometry  Operator=cos
  Trigonometric Function2 : Trigonometry  Operator=cos
  Trigonometric Function3 : Trigonometry
  phi_ddot_numerator : Outport  OutDataTypeStr=double  SampleTime=Tsmall
  wires:
  phi_dot/1 -> Divide1/1, Divide6/3  "phi_dot"
  psi_dot/1 -> Divide4/1, Divide5/4, Divide11/2  "psi_dot"
  Divide6/1 -> Add4/2
  phi/1 -> Divide/1, Trigonometric Function/1, Trigonometric Function1/1  "phi"
  theta/1 -> Trigonometric Function2/1, Trigonometric Function3/1  "theta"
  FY/1 -> Divide2/1  "FY"
  theta_dot/1 -> Divide11/1  "theta_dot"
  Gain2/1 -> Divide/2
  Gain3/1 -> Divide1/2
  Divide1/1 -> Add1/2
  Divide9/1 -> Add2/2
  Divide12/1 -> Add1/3
  Add/1 -> Divide12/1
  Divide3/1 -> Add/2
  Add2/1 -> Divide10/1
  Iyy/1 -> Divide9/2, Add3/1  "Iyy"
  Divide2/1 -> Divide3/1
  Square1/1 -> Divide8/2
  Izz/1 -> Add3/2, Divide8/1  "Izz"
  Add3/1 -> Divide4/2  "del_Iyz"
  Gain/1 -> Add/1
  Add7/1 -> phi_ddot_numerator/1
  Divide8/1 -> Add2/1
  Divide4/1 -> Divide7/1
  Add4/1 -> Divide7/2
  Trigonometric Function2/1 -> Divide3/2, Divide5/3  "cosTheta"
  Divide11/1 -> Divide10/2
  Divide5/1 -> Add4/1
  Divide7/1 -> Add7/2
  Square/1 -> Divide9/1
  Trigonometric Function1/1 -> Divide2/2, Divide5/2, Square/1, Divide6/2  "cosPhi"
  Divide10/1 -> Add7/3
  Add1/1 -> Add7/1
  Trigonometric Function3/1 -> Divide6/4  "sinTheta"
  Divide/1 -> Add1/1
  Trigonometric Function/1 -> Divide5/1, Divide6/1, Square1/1, Gain/1  "sinPhi"
  K_phi/1 -> Gain2/1  "K_phi"
  D_phi/1 -> Gain3/1  "D_phi"
  h/1 -> Divide12/2  "h"
